simulink model "microgridbelbic"  (R2019a)
settings: Solver=VariableStepAuto  StartTime=0.0  StopTime=6  RelTol=1e-3
undefined symbols (not defined in the file): DiscIntNeverNeededParam, fdesignblkfcn, gcbh, Hydride, Metal, Nickel
libraries: powerlib x242, powerlib_extras x28, BELBICtoolbox x4, dsparch4 x1, electricdrivelib x1, simulink x1, sps_avr x1, powerlib_meascontrol x1, re_lib x1
(part 2 of 4)

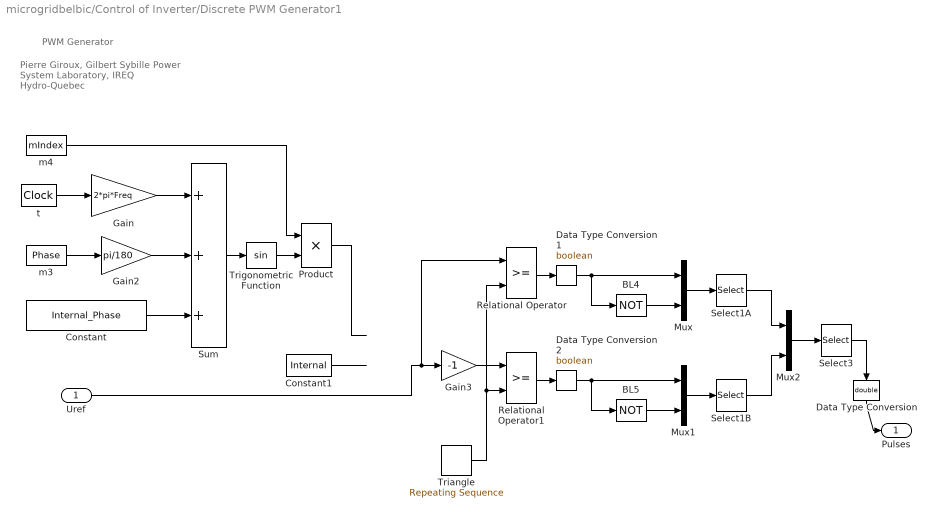
== system microgridbelbic/Control of Inverter/Discrete PWM Generator1 ==
  note: Pierre Giroux, Gilbert Sybille
      | Power System Laboratory, IREQ
      | Hydro-Quebec
  note: PWM Generator
  Uref : Inport
  BL4 : Logic  Operator=NOT  Inputs=1
  BL5 : Logic  Operator=NOT  Inputs=1
  Constant : Constant  Value=Internal_Phase
  Constant1 : Constant  Value=Internal
  Data Type Conversion : DataTypeConversion  OutDataTypeStr=double  SaturateOnIntegerOverflow=on  RndMeth=Zero
  Data Type Conversion1 : DataTypeConversion  OutDataTypeStr=boolean  SaturateOnIntegerOverflow=on  RndMeth=Zero
  Data Type Conversion2 : DataTypeConversion  OutDataTypeStr=boolean  SaturateOnIntegerOverflow=on  RndMeth=Zero
  Gain : Gain  Gain=2*pi*Freq  SaturateOnIntegerOverflow=on  OutDataTypeStr=Inherit: Same as input  ParamDataTypeStr=Inherit: Same as input
  Gain2 : Gain  Gain=pi/180  SaturateOnIntegerOverflow=on  OutDataTypeStr=Inherit: Same as input  ParamDataTypeStr=Inherit: Same as input
  Gain3 : Gain  Gain=-1  SaturateOnIntegerOverflow=on  OutDataTypeStr=Inherit: Same as input  ParamDataTypeStr=Inherit: Same as input
  Mux : Mux  Inputs=2
  Mux1 : Mux  Inputs=2
  Mux2 : Mux  Inputs=2
  Product : Product  SaturateOnIntegerOverflow=on  InputSameDT=on  OutDataTypeStr=Inherit: Same as first input
  Relational Operator : RelationalOperator  RndMeth=Nearest  InputSameDT=on
  Relational Operator1 : RelationalOperator  RndMeth=Nearest  InputSameDT=on
  Select1A : Selector  InputPortWidth=Select1_PortWidth  IndexOptions=Index vector (dialog)  Indices=Select1_Elements  OutputSizes=1
  Select1B : Selector  InputPortWidth=Select1_PortWidth  IndexOptions=Index vector (dialog)  Indices=Select1_Elements  OutputSizes=1
  Select3 : Selector  InputPortWidth=Select3_PortWidth  IndexOptions=Index vector (dialog)  Indices=Select3_Elements  OutputSizes=1
  Sum : Sum  Inputs=+++  SaturateOnIntegerOverflow=on  InputSameDT=on  OutDataTypeStr=Inherit: Same as first input
  Triangle : simulink/Sources/Repeating Sequence  rep_seq_t=[0 1/Fc/4 3/Fc/4 1/Fc]  rep_seq_y=[0 -1 1 0]
  Trigonometric Function : Trigonometry
  m3 : Constant  Value=Phase
  m4 : Constant  Value=mIndex
  t : DigitalClock  SampleTime=Ts
  Pulses : Outport
  wires:
  Mux2/1 -> Select3/1
  Select1B/1 -> Mux2/2
  Select1A/1 -> Mux2/1
  Mux1/1 -> Select1B/1
  Mux/1 -> Select1A/1
  BL5/1 -> Mux1/2
  BL4/1 -> Mux/2
  Gain3/1 -> Relational Operator1/1
  Triangle/1 -> Relational Operator1/2, Relational Operator/2
  Product/1 -> ?
  Constant1/1 -> ?
  Uref/1 -> Relational Operator/1, Gain3/1
  Trigonometric Function/1 -> Product/2
  Sum/1 -> Trigonometric Function/1
  m4/1 -> Product/1
  Constant/1 -> Sum/3
  m3/1 -> Gain2/1
  Gain2/1 -> Sum/2
  Gain/1 -> Sum/1
  t/1 -> Gain/1
  Select3/1 -> Data Type Conversion/1
  Data Type Conversion/1 -> Pulses/1
  Relational Operator/1 -> Data Type Conversion1/1
  Data Type Conversion1/1 -> BL4/1, Mux/1
  Relational Operator1/1 -> Data Type Conversion2/1
  Data Type Conversion2/1 -> BL5/1, Mux1/1

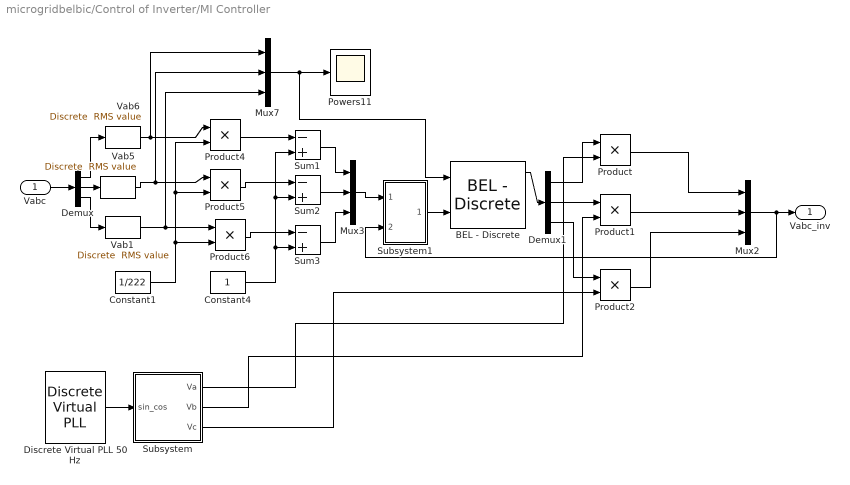
== system microgridbelbic/Control of Inverter/MI Controller ==
  Vabc : Inport
  BEL - Discrete : BELBICtoolbox/Discrete-time/BEL - Discrete  alfa=0.001  beta=0.008  V=0.99  Vth=0.099  W=0.1  T=1
      settings: SourceProductName=BELBIC Toolbox
  Constant1 : Constant  Value=1/222
  Constant4 : Constant
  Demux : Demux  Outputs=3
  Demux1 : Demux  Outputs=3
  Discrete Virtual PLL 50 Hz : powerlib_extras/Discrete  Control Blocks/Discrete Virtual PLL  Freq=50  Phase=0  Ts=20e-6
      settings: SourceProductName=Simscape Electrical  SourceProductBaseCode=PS
  Mux2 : Mux  Inputs=3
  Mux3 : Mux  Inputs=3
  Mux7 : Mux  Inputs=3
  Powers11 : Scope
  Product{,1..2,4..6} (6 alike) : Product  RndMeth=Zero
  Subsystem : Subsystem
  Subsystem1 : Subsystem
  Sum1 : Sum  Inputs=-+  SaturateOnIntegerOverflow=on  InputSameDT=on  OutDataTypeStr=Inherit: Same as first input
  Sum2 : Sum  Inputs=-+  SaturateOnIntegerOverflow=on  InputSameDT=on  OutDataTypeStr=Inherit: Same as first input
  Sum3 : Sum  Inputs=-+  SaturateOnIntegerOverflow=on  InputSameDT=on  OutDataTypeStr=Inherit: Same as first input
  Vab1 : powerlib_extras/Discrete Measurements/Discrete  RMS value  Freq=50  Mag_Init=0  Ts=20e-6
      settings: SourceProductName=Simscape Electrical  SourceProductBaseCode=PS
  Vab5 : powerlib_extras/Discrete Measurements/Discrete  RMS value  Freq=50  Mag_Init=0  Ts=20e-6
      settings: SourceProductName=Simscape Electrical  SourceProductBaseCode=PS
  Vab6 : powerlib_extras/Discrete Measurements/Discrete  RMS value  Freq=50  Mag_Init=0  Ts=20e-6
      settings: SourceProductName=Simscape Electrical  SourceProductBaseCode=PS
  Vabc_inv : Outport
  wires:
  Mux2/1 -> Subsystem1/2(In2), Vabc_inv/1
  Product/1 -> Mux2/1
  Product1/1 -> Mux2/2
  Product2/1 -> Mux2/3
  Vab5/1 -> Mux7/2, Product5/1
  Vab1/1 -> Mux7/3, Product6/1
  Constant4/1 -> Sum3/2, Sum2/2, Sum1/2
  Sum1/1 -> Mux3/1
  Vabc/1 -> Demux/1
  Demux/1 -> Vab6/1
  Demux/2 -> Vab5/1
  Demux/3 -> Vab1/1
  Sum2/1 -> Mux3/2
  Sum3/1 -> Mux3/3
  Demux1/1 -> Product/1
  Demux1/2 -> Product1/1
  Demux1/3 -> Product2/1
  Product4/1 -> Sum1/1
  Product5/1 -> Sum2/1
  Product6/1 -> Sum3/1
  Vab6/1 -> Mux7/1, Product4/1
  Mux7/1 -> BEL - Discrete/1, Powers11/1
  Discrete Virtual PLL 50 Hz/2 -> Subsystem/1(sin_cos)
  Subsystem/1(Va) -> Product/2
  Subsystem/2(Vb) -> Product1/2
  Subsystem/3(Vc) -> Product2/2
  Constant1/1 -> Product6/2, Product5/2, Product4/2
  BEL - Discrete/1 -> Demux1/1
  Mux3/1 -> Subsystem1/1(In1)
  Subsystem1/1(Out1) -> BEL - Discrete/2

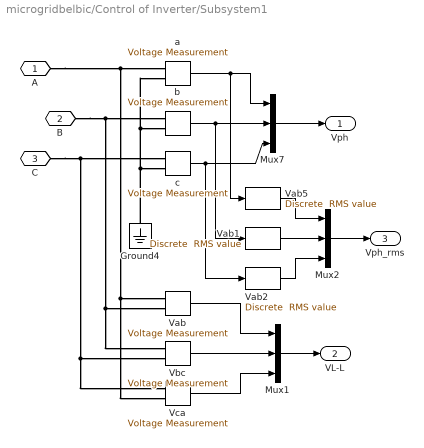
== system microgridbelbic/Control of Inverter/Subsystem1 ==
  Ground4 : powerlib/Elements/Ground  LConnTagsString=a
      settings: SourceProductName=Simscape Electrical
  Mux1 : Mux  Inputs=3
  Mux2 : Mux  Inputs=3
  Mux7 : Mux  Inputs=3
  Vab : powerlib/Measurements/Voltage Measurement  Tag=PoWeRsYsTeMmEaSuReMeNt  PhasorSimulation=off  OutputType=Magnitude  PSBequivalent=0
      settings: SourceProductName=Simscape Electrical
  Vab1 : powerlib_extras/Discrete Measurements/Discrete  RMS value  Freq=50  Mag_Init=0  Ts=20e-6
      settings: SourceProductName=Simscape Electrical  SourceProductBaseCode=PS
  Vab2 : powerlib_extras/Discrete Measurements/Discrete  RMS value  Freq=50  Mag_Init=0  Ts=20e-6
      settings: SourceProductName=Simscape Electrical  SourceProductBaseCode=PS
  Vab5 : powerlib_extras/Discrete Measurements/Discrete  RMS value  Freq=50  Mag_Init=0  Ts=20e-6
      settings: SourceProductName=Simscape Electrical  SourceProductBaseCode=PS
  Vbc : powerlib/Measurements/Voltage Measurement  Tag=PoWeRsYsTeMmEaSuReMeNt  PhasorSimulation=off  OutputType=Magnitude  PSBequivalent=0
      settings: SourceProductName=Simscape Electrical
  Vca : powerlib/Measurements/Voltage Measurement  Tag=PoWeRsYsTeMmEaSuReMeNt  PhasorSimulation=off  OutputType=Magnitude  PSBequivalent=0
      settings: SourceProductName=Simscape Electrical
  a : powerlib/Measurements/Voltage Measurement  Tag=PoWeRsYsTeMmEaSuReMeNt  PhasorSimulation=off  OutputType=Magnitude  PSBequivalent=0
      settings: SourceProductName=Simscape Electrical
  b : powerlib/Measurements/Voltage Measurement  Tag=PoWeRsYsTeMmEaSuReMeNt  PhasorSimulation=off  OutputType=Magnitude  PSBequivalent=0
      settings: SourceProductName=Simscape Electrical
  c : powerlib/Measurements/Voltage Measurement  Tag=PoWeRsYsTeMmEaSuReMeNt  PhasorSimulation=off  OutputType=Magnitude  PSBequivalent=0
      settings: SourceProductName=Simscape Electrical
  A : PMIOPort  Side=Left
  B : PMIOPort  Port=2  Side=Left
  C : PMIOPort  Port=3  Side=Left
  Vph : Outport
  VL-L : Outport  Port=2
  Vph_rms : Outport  Port=3
  wires:
  a/1 -> Mux7/1, Vab5/1
  b/1 -> Mux7/2, Vab1/1
  c/1 -> Mux7/3, Vab2/1
  Mux7/1 -> Vph/1
  Vab/1 -> Mux1/1
  Vbc/1 -> Mux1/2
  Vca/1 -> Mux1/3
  Mux1/1 -> VL-L/1
  Vab5/1 -> Mux2/1
  Vab1/1 -> Mux2/2
  Vab2/1 -> Mux2/3
  Mux2/1 -> Vph_rms/1
  connections:
  Ground4/LConn1 -- c/LConn2 -- b/LConn2 -- a/LConn2
  A/RConn1 -- a/LConn1 -- Vab/LConn1 -- Vca/LConn2
  B/RConn1 -- b/LConn1 -- Vab/LConn2 -- Vbc/LConn1
  C/RConn1 -- c/LConn1 -- Vbc/LConn2 -- Vca/LConn1

== system microgridbelbic/Diesel/Diesel Engine Speed & Voltage Control ==
  wref : Inport
  Vtref : Inport  Port=2
  m : Inport  Port=3
  Bus Selector : BusSelector  OutputSignals="Mechanical.Rotor speed  wm  (pu)"
  Bus Selector1 : BusSelector  OutputSignals="dq0 components.Stator voltage  vd (pu),dq0 components.Stator voltage  vq (pu)"  OutputAsBus=on
  Demux2 : Demux  Outputs=2
  EXCITATION : sps_avr/Excitation System  tr=20e-3  reg=[ 200, 0.02 ]  exc=[ 1, 0 ]  tgr=[ 0, 0 ]  damp=[ 0.001, 0.1 ]  sat=[ 0, 0 ]  lim=[ 0, 6, 0 ]  v0=[1,1.42734]
      settings: SourceProductName=Simscape Electrical  SourceProductBaseCode=PS
  Fcn : Fcn  Expr=sqrt(u(1)^2 + u(2)^2)
  GOVERNOR & DIESEL ENGINE : Subsystem  mask(Diesel Engine & Governor){K=40, Tr=[0.01 0.02 0.2], Ta=[0.25 0.009 0.0384], Tlim=[0 1.1], Td=0.024, Pm0=0.000270147}
      mask prompts: K "Regulator gain K:"; Tr "Regulator time constants [T1 T2 T3 ] (s) :"; Ta "Actuator time constants [T4 T5 T6] (s) :"; Tlim "Torque limits [Tmin Tmax] (pu) :"; Td "Engine time delay Td (s) :"; Pm0 "Initial value of mechanical power  Pm0 (pu) :"
      mask help:
      | This block implements a diesel engine and governor system:
      | 1st and 2nd inputs: Desired and actual speed (pu)
      | Output: Diesel engine mechanical power.Motor inertia should be combined with generator.
      | Controller transfer function:
      |      Hc=K.(1+T3.s)/(1+T1.s+T1.T2.s^2)
      | Actuator transfer function :
      |      Ha= (1+T4.s) / [ (s (1+T5.s)(1+T6.s) ]
      | Motor :
      |      Time delay Td
      |
      | (See reference in Tutorial Session 5)
  Ground : Ground
  Pm : Outport  InitialOutput=0
  Vf : Outport  Port=2  InitialOutput=0
  Vt : Outport  Port=3  InitialOutput=0
  w : Outport  Port=4  InitialOutput=0
  wires:
  Ground/1 -> EXCITATION/4
  m/1 -> Bus Selector/1, Bus Selector1/1
  wref/1 -> GOVERNOR & DIESEL ENGINE/1(wref (pu))
  Demux2/2 -> EXCITATION/3
  EXCITATION/1 -> Vf/1
  GOVERNOR & DIESEL ENGINE/1(Pmec (pu)) -> Pm/1
  Vtref/1 -> EXCITATION/1
  Demux2/1 -> EXCITATION/2
  Bus Selector1/1 -> Demux2/1, Fcn/1
  Fcn/1 -> Vt/1
  Bus Selector/1 -> GOVERNOR & DIESEL ENGINE/2(w (pu)), w/1  "<Rotor speed  wm  (pu)>"

== system microgridbelbic/Subsystem/Subsystem ==
  In1 : Inport
  In2 : Inport  Port=2
  Add : Sum
  Gain1 : Gain  Gain=0.02
  Gain2 : Gain  Gain=0.001
  Out1 : Outport
  wires:
  In1/1 -> Gain1/1
  Gain2/1 -> Add/2
  In2/1 -> Gain2/1
  Add/1 -> Out1/1
  Gain1/1 -> Add/1

== system microgridbelbic/Subsystem1/Subsystem ==
  In1 : Inport
  array1 : Subsystem
  array6 : Subsystem
  array7 : Subsystem
  Conn3 : PMIOPort  Side=Right
  Conn4 : PMIOPort  Port=2  Side=Right
  wires:
  In1/1 -> array1/1(In1), array7/1(In1), array6/1(In1)
  connections:
  array1/RConn2 -- array6/RConn2 -- array7/RConn2 -- Conn4/RConn1
  array1/RConn1 -- array6/RConn1 -- array7/RConn1 -- Conn3/RConn1

== system microgridbelbic/Subsystem1/Subsystem1 ==
  In1 : Inport
  array1 : Subsystem
  array6 : Subsystem
  array7 : Subsystem
  Conn3 : PMIOPort  Side=Right
  Conn4 : PMIOPort  Port=2  Side=Right
  wires:
  In1/1 -> array1/1(In1), array7/1(In1), array6/1(In1)
  connections:
  array1/RConn1 -- array7/RConn1 -- array6/RConn1 -- Conn3/RConn1
  array1/RConn2 -- array7/RConn2 -- array6/RConn2 -- Conn4/RConn1

== system microgridbelbic/Subsystem1/Subsystem2 ==
  In1 : Inport
  array1 : Subsystem
  array6 : Subsystem
  array7 : Subsystem
  Conn3 : PMIOPort  Side=Right
  Conn4 : PMIOPort  Port=2  Side=Right
  wires:
  In1/1 -> array1/1(In1), array7/1(In1), array6/1(In1)
  connections:
  array1/RConn2 -- array7/RConn2 -- array6/RConn2 -- Conn4/RConn1
  array1/RConn1 -- array7/RConn1 -- array6/RConn1 -- Conn3/RConn1

== system microgridbelbic/Subsystem1/Subsystem3 ==
  In1 : Inport
  array1 : Subsystem
  array6 : Subsystem
  array7 : Subsystem
  Conn3 : PMIOPort  Side=Right
  Conn4 : PMIOPort  Port=2  Side=Right
  wires:
  In1/1 -> array1/1(In1), array7/1(In1), array6/1(In1)
  connections:
  array1/RConn2 -- array7/RConn2 -- array6/RConn2 -- Conn4/RConn1
  array1/RConn1 -- array7/RConn1 -- array6/RConn1 -- Conn3/RConn1

== system microgridbelbic/Subsystem1/Subsystem4 ==
  In1 : Inport
  array1 : Subsystem
  array6 : Subsystem
  array7 : Subsystem
  Conn3 : PMIOPort  Side=Right
  Conn4 : PMIOPort  Port=2  Side=Right
  wires:
  In1/1 -> array1/1(In1), array7/1(In1), array6/1(In1)
  connections:
  array1/RConn1 -- array7/RConn1 -- Conn3/RConn1 -- array6/RConn1
  array1/RConn2 -- array7/RConn2 -- Conn4/RConn1 -- array6/RConn2

== system microgridbelbic/Wind pulses/Current Controller1 ==
  Iref : Inport
  Ia : Inport  Port=2
  Relay : Relay  OnSwitchValue=h/2  OffSwitchValue=-h/2
  Sum1 : Sum  Inputs=-+  SaturateOnIntegerOverflow=on  InputSameDT=on  OutDataTypeStr=Inherit: Same as first input
  g : Outport  InitialOutput=0
  error1 : Outport  Port=2  InitialOutput=0
  wires:
  Sum1/1 -> error1/1, Relay/1
  Iref/1 -> Sum1/2
  Ia/1 -> Sum1/1
  Relay/1 -> g/1

== system microgridbelbic/Wind pulses/Subsystem ==
  Tref : Inport
  wm : Inport  Port=2
  Vd : Inport  Port=3
  Avoid division by zero : Saturate  UpperLimit=1e6  LowerLimit=1e-6
  Base Torque1 : Product  Inputs=*/  RndMeth=Zero
  Product1 : Product  RndMeth=Zero
  Id_ref : Outport
  wires:
  Vd/1 -> Avoid division by zero/1
  Base Torque1/1 -> Id_ref/1
  wm/1 -> Product1/2
  Tref/1 -> Product1/1
  Avoid division by zero/1 -> Base Torque1/2
  Product1/1 -> Base Torque1/1

== system microgridbelbic/Wind pulses/Torque reference 1 ==
  wm : Inport
  1\ib1 : Gain  Gain=0.001189  SaturateOnIntegerOverflow=on  OutDataTypeStr=Inherit: Same as input  ParamDataTypeStr=Inherit: Same as input
  1\ib2 : Gain  Gain=0.0197  SaturateOnIntegerOverflow=on  OutDataTypeStr=Inherit: Same as input  ParamDataTypeStr=Inherit: Same as input
  Add : Sum
  Constant2 : Constant  Value=1.791e-3
  Differentiator Filter : Subsystem  DialogController=fdesignblkfcn  InitFcn=fdesignblkfcn(gcbh, {'InitFcn'});  mask(Differentiator Filter){}
      mask help: Design a differentiator filter
      settings: CopyFcn=fdesignblkfcn(gcbh, {'CopyFcn'});
      mask Help: helpview(mapfilelocation('dspblks'), 'dspdifferentiatorfilter')
      mask Display: disp('Differentiator');
  Math Function : Math  Operator=square  SaturateOnIntegerOverflow=on
  Product1 : Product  RndMeth=Zero
  Ref. sat.1 : Saturate  UpperLimit=inf  LowerLimit=0
  Subtract : Sum  Inputs=+-
  Tref : Outport
  wires:
  Subtract/1 -> Ref. sat.1/1
  1\ib2/1 -> Add/1
  Product1/1 -> Subtract/1
  1\ib1/1 -> Add/2
  Differentiator Filter/1(Out) -> 1\ib2/1
  Ref. sat.1/1 -> Tref/1
  wm/1 -> 1\ib1/1, Differentiator Filter/1(In), Math Function/1
  Constant2/1 -> Product1/2
  Math Function/1 -> Product1/1

== system microgridbelbic/wind1 20.1KW/Pitch_angle-controller ==
  wr : Inport
  0-pitch_max : Saturate  UpperLimit=45  LowerLimit=0
  Constant2 : Constant
  "Rate Limiter   " : RateLimiter  RisingSlewLimit=2  FallingSlewLimit=-2
  Sum : Sum  Inputs=|+-  SaturateOnIntegerOverflow=on
  genertaor terminal6 : Scope  NumInputPorts=2
  pitch_gain : Gain  Gain=500  SaturateOnIntegerOverflow=on  OutDataTypeStr=Inherit: Same as input  ParamDataTypeStr=Inherit: Same as input
  Pitch_angle : Outport
  wires:
  wr/1 -> Sum/1
  0-pitch_max/1 -> genertaor terminal6/2, "Rate Limiter   "/1
  Constant2/1 -> Sum/2
  Sum/1 -> pitch_gain/1
  pitch_gain/1 -> 0-pitch_max/1
  "Rate Limiter   "/1 -> genertaor terminal6/1, Pitch_angle/1

== system microgridbelbic/Control of Inverter/MI Controller/Subsystem ==
  sin_cos : Inport  PortDimensions=2
  Demux : Demux  Outputs=2
  Fcn2 : Fcn  Expr=1*u[1]
  Fcn4 : Fcn  Expr=1*u[3]
  Fcn5 : Fcn  Expr=1*u[5]
  K1 : Constant  Value=0.5
  K2 : Constant  Value=sqrt(3)/2
  Mux2 : Mux  Inputs=6
  Product{,1..3} (4 alike) : Product  SaturateOnIntegerOverflow=on  InputSameDT=on  OutDataTypeStr=Inherit: Same as first input
  Sum : Sum  Inputs=--  SaturateOnIntegerOverflow=on  InputSameDT=on  OutDataTypeStr=Inherit: Same as first input
  Sum1 : Sum  Inputs=-+  SaturateOnIntegerOverflow=on  InputSameDT=on  OutDataTypeStr=Inherit: Same as first input
  Sum2 : Sum  Inputs=--  SaturateOnIntegerOverflow=on  InputSameDT=on  OutDataTypeStr=Inherit: Same as first input
  Sum3 : Sum  Inputs=--  SaturateOnIntegerOverflow=on  InputSameDT=on  OutDataTypeStr=Inherit: Same as first input
  Va : Outport
  Vb : Outport  Port=2
  Vc : Outport  Port=3
  wires:
  sin_cos/1 -> Demux/1
  Demux/1 -> Product/1, Product2/1, Sum2/2, Mux2/1  "sin(wt)"
  Product/1 -> Sum/1
  Product1/1 -> Sum/2
  Product3/1 -> Sum1/1
  Product2/1 -> Sum1/2
  Sum3/1 -> Mux2/6  "cos(wt+2pi/3)"
  Sum2/1 -> Mux2/5  "sin(wt+2pi/3)"
  K1/1 -> Product/2, Product3/2
  K2/1 -> Product1/2, Product2/2
  Sum/1 -> Mux2/3, Sum2/1  "sin(wt-2pi/3)"
  Sum1/1 -> Mux2/4, Sum3/1  "cos(wt-2pi/3)"
  Demux/2 -> Sum3/2, Product3/1, Product1/1, Mux2/2  "cos(wt)"
  Mux2/1 -> Fcn2/1, Fcn4/1, Fcn5/1
  Fcn2/1 -> Va/1
  Fcn4/1 -> Vb/1
  Fcn5/1 -> Vc/1

== system microgridbelbic/Control of Inverter/MI Controller/Subsystem1 ==
  In1 : Inport
  In2 : Inport  Port=2
  Add : Sum
  Gain1 : Gain  Gain=0.9
  Gain2 : Gain  Gain=0.01
  Out1 : Outport
  wires:
  In1/1 -> Gain1/1
  Gain2/1 -> Add/2
  In2/1 -> Gain2/1
  Add/1 -> Out1/1
  Gain1/1 -> Add/1

== system microgridbelbic/Diesel/Diesel Engine Speed & Voltage Control/GOVERNOR & DIESEL ENGINE ==
  note: ACTUATOR
  wref (pu) : Inport
  w (pu) : Inport  Port=2
  CONTROL SYSTEM : TransferFcn  Numerator=([Tr(3) 1])  Denominator="([Tr(1)*Tr(2)  Tr(1) 1])"
  ENGINE Td : TransportDelay  DelayTime=Td  InitialOutput=Pm0
  Gain K : Gain  Gain=K  SaturateOnIntegerOverflow=on  OutDataTypeStr=Inherit: Same as input  ParamDataTypeStr=Inherit: Same as input
  Integrator : Integrator  InitialCondition=Pm0  LimitOutput=on  UpperSaturationLimit=Tlim(2)  LowerSaturationLimit=Tlim(1)
  Product : Product  SaturateOnIntegerOverflow=on  InputSameDT=on  OutDataTypeStr=Inherit: Same as first input
  Sum : Sum  Inputs=+-  SaturateOnIntegerOverflow=on  InputSameDT=on  OutDataTypeStr=Inherit: Same as first input
  TF1 : TransferFcn  Numerator=([Ta(1) 1])  Denominator=([Ta(2) 1])
  TF2 : TransferFcn  Numerator=1  Denominator=([Ta(3) 1])
  Pmec (pu) : Outport  InitialOutput=0
  wires:
  Gain K/1 -> TF1/1
  Sum/1 -> CONTROL SYSTEM/1
  CONTROL SYSTEM/1 -> Gain K/1
  TF1/1 -> TF2/1
  w (pu)/1 -> Product/2, Sum/2
  ENGINE Td/1 -> Product/1
  wref (pu)/1 -> Sum/1
  Product/1 -> Pmec (pu)/1
  TF2/1 -> Integrator/1
  Integrator/1 -> ENGINE Td/1  "Torque"

== system microgridbelbic/Subsystem1/Subsystem/array1 ==
  In1 : Inport
  Solar : Subsystem
  Conn1 : PMIOPort  Side=Right
  Conn2 : PMIOPort  Port=2  Side=Right
  wires:
  In1/1 -> Solar/1(In1)
  connections:
  Solar/RConn1 -- Conn1/RConn1
  Solar/RConn3 -- Solar/RConn2
  Conn2/RConn1 -- Solar/RConn4

== system microgridbelbic/Subsystem1/Subsystem/array6 ==
  In1 : Inport
  Solar : Subsystem
  Conn1 : PMIOPort  Side=Right
  Conn2 : PMIOPort  Port=2  Side=Right
  wires:
  In1/1 -> Solar/1(In1)
  connections:
  Conn2/RConn1 -- Solar/RConn4
  Solar/RConn3 -- Solar/RConn2
  Solar/RConn1 -- Conn1/RConn1

== system microgridbelbic/Subsystem1/Subsystem/array7 ==
  In1 : Inport
  Solar : Subsystem
  Conn1 : PMIOPort  Side=Right
  Conn2 : PMIOPort  Port=2  Side=Right
  wires:
  In1/1 -> Solar/1(In1)
  connections:
  Conn2/RConn1 -- Solar/RConn4
  Solar/RConn3 -- Solar/RConn2
  Solar/RConn1 -- Conn1/RConn1

== system microgridbelbic/Subsystem1/Subsystem1/array1 ==
  In1 : Inport
  Solar : Subsystem
  Conn1 : PMIOPort  Side=Right
  Conn2 : PMIOPort  Port=2  Side=Right
  wires:
  In1/1 -> Solar/1(In1)
  connections:
  Conn2/RConn1 -- Solar/RConn4
  Solar/RConn3 -- Solar/RConn2
  Solar/RConn1 -- Conn1/RConn1

== system microgridbelbic/Subsystem1/Subsystem1/array6 ==
  In1 : Inport
  Solar : Subsystem
  Conn1 : PMIOPort  Side=Right
  Conn2 : PMIOPort  Port=2  Side=Right
  wires:
  In1/1 -> Solar/1(In1)
  connections:
  Solar/RConn1 -- Conn1/RConn1
  Solar/RConn3 -- Solar/RConn2
  Conn2/RConn1 -- Solar/RConn4

== system microgridbelbic/Subsystem1/Subsystem1/array7 ==
  In1 : Inport
  Solar : Subsystem
  Conn1 : PMIOPort  Side=Right
  Conn2 : PMIOPort  Port=2  Side=Right
  wires:
  In1/1 -> Solar/1(In1)
  connections:
  Solar/RConn1 -- Conn1/RConn1
  Solar/RConn3 -- Solar/RConn2
  Conn2/RConn1 -- Solar/RConn4

== system microgridbelbic/Subsystem1/Subsystem2/array1 ==
  In1 : Inport
  Solar : Subsystem
  Conn1 : PMIOPort  Side=Right
  Conn2 : PMIOPort  Port=2  Side=Right
  wires:
  In1/1 -> Solar/1(In1)
  connections:
  Solar/RConn1 -- Conn1/RConn1
  Solar/RConn3 -- Solar/RConn2
  Conn2/RConn1 -- Solar/RConn4

== system microgridbelbic/Subsystem1/Subsystem2/array6 ==
  In1 : Inport
  Solar : Subsystem
  Conn1 : PMIOPort  Side=Right
  Conn2 : PMIOPort  Port=2  Side=Right
  wires:
  In1/1 -> Solar/1(In1)
  connections:
  Conn2/RConn1 -- Solar/RConn4
  Solar/RConn3 -- Solar/RConn2
  Solar/RConn1 -- Conn1/RConn1

== system microgridbelbic/Subsystem1/Subsystem2/array7 ==
  In1 : Inport
  Solar : Subsystem
  Conn1 : PMIOPort  Side=Right
  Conn2 : PMIOPort  Port=2  Side=Right
  wires:
  In1/1 -> Solar/1(In1)
  connections:
  Conn2/RConn1 -- Solar/RConn4
  Solar/RConn3 -- Solar/RConn2
  Solar/RConn1 -- Conn1/RConn1

== system microgridbelbic/Subsystem1/Subsystem3/array1 ==
  In1 : Inport
  Solar : Subsystem
  Conn1 : PMIOPort  Side=Right
  Conn2 : PMIOPort  Port=2  Side=Right
  wires:
  In1/1 -> Solar/1(In1)
  connections:
  Solar/RConn1 -- Conn1/RConn1
  Solar/RConn3 -- Solar/RConn2
  Conn2/RConn1 -- Solar/RConn4

== system microgridbelbic/Subsystem1/Subsystem3/array6 ==
  In1 : Inport
  Solar : Subsystem
  Conn1 : PMIOPort  Side=Right
  Conn2 : PMIOPort  Port=2  Side=Right
  wires:
  In1/1 -> Solar/1(In1)
  connections:
  Conn2/RConn1 -- Solar/RConn4
  Solar/RConn3 -- Solar/RConn2
  Solar/RConn1 -- Conn1/RConn1

== system microgridbelbic/Subsystem1/Subsystem3/array7 ==
  In1 : Inport
  Solar : Subsystem
  Conn1 : PMIOPort  Side=Right
  Conn2 : PMIOPort  Port=2  Side=Right
  wires:
  In1/1 -> Solar/1(In1)
  connections:
  Conn2/RConn1 -- Solar/RConn4
  Solar/RConn3 -- Solar/RConn2
  Solar/RConn1 -- Conn1/RConn1

== system microgridbelbic/Subsystem1/Subsystem4/array1 ==
  In1 : Inport
  Solar : Subsystem
  Conn1 : PMIOPort  Side=Right
  Conn2 : PMIOPort  Port=2  Side=Right
  wires:
  In1/1 -> Solar/1(In1)
  connections:
  Conn2/RConn1 -- Solar/RConn4
  Solar/RConn3 -- Solar/RConn2
  Solar/RConn1 -- Conn1/RConn1

== system microgridbelbic/Subsystem1/Subsystem4/array6 ==
  In1 : Inport
  Solar : Subsystem
  Conn1 : PMIOPort  Side=Right
  Conn2 : PMIOPort  Port=2  Side=Right
  wires:
  In1/1 -> Solar/1(In1)
  connections:
  Solar/RConn1 -- Conn1/RConn1
  Solar/RConn3 -- Solar/RConn2
  Conn2/RConn1 -- Solar/RConn4

== system microgridbelbic/Subsystem1/Subsystem4/array7 ==
  In1 : Inport
  Solar : Subsystem
  Conn1 : PMIOPort  Side=Right
  Conn2 : PMIOPort  Port=2  Side=Right
  wires:
  In1/1 -> Solar/1(In1)
  connections:
  Solar/RConn1 -- Conn1/RConn1
  Solar/RConn3 -- Solar/RConn2
  Conn2/RConn1 -- Solar/RConn4

== system microgridbelbic/Wind pulses/Torque reference 1/Differentiator Filter ==
  In : Inport
  Generated Filter Block : Subsystem  Tag=FilterWizardSubSystem
      settings: ErrorFcn=dspFilterRealizedInBasicElemsAlgLoopErrFcnCallback
  Out : Outport
  wires:
  In/1 -> Generated Filter Block/1(Input)
  Generated Filter Block/1(Output) -> Out/1

== system microgridbelbic/Subsystem1/Subsystem/array1/Solar ==
  In1 : Inport
  Subsystem1 : Subsystem
  Subsystem5 : Subsystem
  1 : PMIOPort  Tag=PMCPort  Side=Right
  2 : PMIOPort  Tag=PMCPort  Port=2  Side=Right
  3 : PMIOPort  Tag=PMCPort  Port=3  Side=Right
  4 : PMIOPort  Tag=PMCPort  Port=4  Side=Right
  wires:
  In1/1 -> Subsystem1/1(In1), Subsystem5/1(In1)
  connections:
  3/RConn1 -- Subsystem1/RConn1
  4/RConn1 -- Subsystem1/RConn2
  1/RConn1 -- Subsystem5/RConn1
  2/RConn1 -- Subsystem5/RConn2

== system microgridbelbic/Subsystem1/Subsystem/array6/Solar ==
  In1 : Inport
  "11= Vmpp=336V, Voc=406V" : Subsystem
  "11=336V, 406 V" : Subsystem
  1 : PMIOPort  Tag=PMCPort  Side=Right
  2 : PMIOPort  Tag=PMCPort  Port=2  Side=Right
  3 : PMIOPort  Tag=PMCPort  Port=3  Side=Right
  4 : PMIOPort  Tag=PMCPort  Port=4  Side=Right
  wires:
  In1/1 -> "11= Vmpp=336V, Voc=406V"/1(In1), "11=336V, 406 V"/1(In1)
  connections:
  2/RConn1 -- "11= Vmpp=336V, Voc=406V"/RConn2
  1/RConn1 -- "11= Vmpp=336V, Voc=406V"/RConn1
  4/RConn1 -- "11=336V, 406 V"/RConn2
  3/RConn1 -- "11=336V, 406 V"/RConn1

== system microgridbelbic/Subsystem1/Subsystem/array7/Solar ==
  In1 : Inport
  Subsystem1 : Subsystem
  Subsystem5 : Subsystem
  1 : PMIOPort  Tag=PMCPort  Side=Right
  2 : PMIOPort  Tag=PMCPort  Port=2  Side=Right
  3 : PMIOPort  Tag=PMCPort  Port=3  Side=Right
  4 : PMIOPort  Tag=PMCPort  Port=4  Side=Right
  wires:
  In1/1 -> Subsystem5/1(In1), Subsystem1/1(In1)
  connections:
  2/RConn1 -- Subsystem5/RConn2
  1/RConn1 -- Subsystem5/RConn1
  4/RConn1 -- Subsystem1/RConn2
  3/RConn1 -- Subsystem1/RConn1

== system microgridbelbic/Subsystem1/Subsystem1/array1/Solar ==
  In1 : Inport
  Subsystem1 : Subsystem
  Subsystem5 : Subsystem
  1 : PMIOPort  Tag=PMCPort  Side=Right
  2 : PMIOPort  Tag=PMCPort  Port=2  Side=Right
  3 : PMIOPort  Tag=PMCPort  Port=3  Side=Right
  4 : PMIOPort  Tag=PMCPort  Port=4  Side=Right
  wires:
  In1/1 -> Subsystem5/1(In1), Subsystem1/1(In1)
  connections:
  2/RConn1 -- Subsystem5/RConn2
  1/RConn1 -- Subsystem5/RConn1
  4/RConn1 -- Subsystem1/RConn2
  3/RConn1 -- Subsystem1/RConn1

== system microgridbelbic/Subsystem1/Subsystem1/array6/Solar ==
  In1 : Inport
  "11= Vmpp=336V, Voc=406V" : Subsystem
  "11=336V, 406 V" : Subsystem
  1 : PMIOPort  Tag=PMCPort  Side=Right
  2 : PMIOPort  Tag=PMCPort  Port=2  Side=Right
  3 : PMIOPort  Tag=PMCPort  Port=3  Side=Right
  4 : PMIOPort  Tag=PMCPort  Port=4  Side=Right
  wires:
  In1/1 -> "11=336V, 406 V"/1(In1), "11= Vmpp=336V, Voc=406V"/1(In1)
  connections:
  3/RConn1 -- "11=336V, 406 V"/RConn1
  4/RConn1 -- "11=336V, 406 V"/RConn2
  1/RConn1 -- "11= Vmpp=336V, Voc=406V"/RConn1
  2/RConn1 -- "11= Vmpp=336V, Voc=406V"/RConn2

== system microgridbelbic/Subsystem1/Subsystem1/array7/Solar ==
  In1 : Inport
  Subsystem1 : Subsystem
  Subsystem5 : Subsystem
  1 : PMIOPort  Tag=PMCPort  Side=Right
  2 : PMIOPort  Tag=PMCPort  Port=2  Side=Right
  3 : PMIOPort  Tag=PMCPort  Port=3  Side=Right
  4 : PMIOPort  Tag=PMCPort  Port=4  Side=Right
  wires:
  In1/1 -> Subsystem1/1(In1), Subsystem5/1(In1)
  connections:
  3/RConn1 -- Subsystem1/RConn1
  4/RConn1 -- Subsystem1/RConn2
  1/RConn1 -- Subsystem5/RConn1
  2/RConn1 -- Subsystem5/RConn2

== system microgridbelbic/Subsystem1/Subsystem2/array1/Solar ==
  In1 : Inport
  Subsystem1 : Subsystem
  Subsystem5 : Subsystem
  1 : PMIOPort  Tag=PMCPort  Side=Right
  2 : PMIOPort  Tag=PMCPort  Port=2  Side=Right
  3 : PMIOPort  Tag=PMCPort  Port=3  Side=Right
  4 : PMIOPort  Tag=PMCPort  Port=4  Side=Right
  wires:
  In1/1 -> Subsystem1/1(In1), Subsystem5/1(In1)
  connections:
  3/RConn1 -- Subsystem1/RConn1
  4/RConn1 -- Subsystem1/RConn2
  1/RConn1 -- Subsystem5/RConn1
  2/RConn1 -- Subsystem5/RConn2

== system microgridbelbic/Subsystem1/Subsystem2/array6/Solar ==
  In1 : Inport
  "11= Vmpp=336V, Voc=406V" : Subsystem
  "11=336V, 406 V" : Subsystem
  1 : PMIOPort  Tag=PMCPort  Side=Right
  2 : PMIOPort  Tag=PMCPort  Port=2  Side=Right
  3 : PMIOPort  Tag=PMCPort  Port=3  Side=Right
  4 : PMIOPort  Tag=PMCPort  Port=4  Side=Right
  wires:
  In1/1 -> "11= Vmpp=336V, Voc=406V"/1(In1), "11=336V, 406 V"/1(In1)
  connections:
  2/RConn1 -- "11= Vmpp=336V, Voc=406V"/RConn2
  1/RConn1 -- "11= Vmpp=336V, Voc=406V"/RConn1
  4/RConn1 -- "11=336V, 406 V"/RConn2
  3/RConn1 -- "11=336V, 406 V"/RConn1

== system microgridbelbic/Subsystem1/Subsystem2/array7/Solar ==
  In1 : Inport
  Subsystem1 : Subsystem
  Subsystem5 : Subsystem
  1 : PMIOPort  Tag=PMCPort  Side=Right
  2 : PMIOPort  Tag=PMCPort  Port=2  Side=Right
  3 : PMIOPort  Tag=PMCPort  Port=3  Side=Right
  4 : PMIOPort  Tag=PMCPort  Port=4  Side=Right
  wires:
  In1/1 -> Subsystem5/1(In1), Subsystem1/1(In1)
  connections:
  2/RConn1 -- Subsystem5/RConn2
  1/RConn1 -- Subsystem5/RConn1
  4/RConn1 -- Subsystem1/RConn2
  3/RConn1 -- Subsystem1/RConn1

== system microgridbelbic/Subsystem1/Subsystem3/array1/Solar ==
  In1 : Inport
  Subsystem1 : Subsystem
  Subsystem5 : Subsystem
  1 : PMIOPort  Tag=PMCPort  Side=Right
  2 : PMIOPort  Tag=PMCPort  Port=2  Side=Right
  3 : PMIOPort  Tag=PMCPort  Port=3  Side=Right
  4 : PMIOPort  Tag=PMCPort  Port=4  Side=Right
  wires:
  In1/1 -> Subsystem1/1(In1), Subsystem5/1(In1)
  connections:
  3/RConn1 -- Subsystem1/RConn1
  4/RConn1 -- Subsystem1/RConn2
  1/RConn1 -- Subsystem5/RConn1
  2/RConn1 -- Subsystem5/RConn2

== system microgridbelbic/Subsystem1/Subsystem3/array6/Solar ==
  In1 : Inport
  "11= Vmpp=336V, Voc=406V" : Subsystem
  "11=336V, 406 V" : Subsystem
  1 : PMIOPort  Tag=PMCPort  Side=Right
  2 : PMIOPort  Tag=PMCPort  Port=2  Side=Right
  3 : PMIOPort  Tag=PMCPort  Port=3  Side=Right
  4 : PMIOPort  Tag=PMCPort  Port=4  Side=Right
  wires:
  In1/1 -> "11= Vmpp=336V, Voc=406V"/1(In1), "11=336V, 406 V"/1(In1)
  connections:
  2/RConn1 -- "11= Vmpp=336V, Voc=406V"/RConn2
  1/RConn1 -- "11= Vmpp=336V, Voc=406V"/RConn1
  4/RConn1 -- "11=336V, 406 V"/RConn2
  3/RConn1 -- "11=336V, 406 V"/RConn1

== system microgridbelbic/Subsystem1/Subsystem3/array7/Solar ==
  In1 : Inport
  Subsystem1 : Subsystem
  Subsystem5 : Subsystem
  1 : PMIOPort  Tag=PMCPort  Side=Right
  2 : PMIOPort  Tag=PMCPort  Port=2  Side=Right
  3 : PMIOPort  Tag=PMCPort  Port=3  Side=Right
  4 : PMIOPort  Tag=PMCPort  Port=4  Side=Right
  wires:
  In1/1 -> Subsystem5/1(In1), Subsystem1/1(In1)
  connections:
  2/RConn1 -- Subsystem5/RConn2
  1/RConn1 -- Subsystem5/RConn1
  4/RConn1 -- Subsystem1/RConn2
  3/RConn1 -- Subsystem1/RConn1

== system microgridbelbic/Subsystem1/Subsystem4/array1/Solar ==
  In1 : Inport
  Subsystem1 : Subsystem
  Subsystem5 : Subsystem
  1 : PMIOPort  Tag=PMCPort  Side=Right
  2 : PMIOPort  Tag=PMCPort  Port=2  Side=Right
  3 : PMIOPort  Tag=PMCPort  Port=3  Side=Right
  4 : PMIOPort  Tag=PMCPort  Port=4  Side=Right
  wires:
  In1/1 -> Subsystem5/1(In1), Subsystem1/1(In1)
  connections:
  2/RConn1 -- Subsystem5/RConn2
  1/RConn1 -- Subsystem5/RConn1
  4/RConn1 -- Subsystem1/RConn2
  3/RConn1 -- Subsystem1/RConn1

== system microgridbelbic/Subsystem1/Subsystem4/array6/Solar ==
  In1 : Inport
  "11= Vmpp=336V, Voc=406V" : Subsystem
  "11=336V, 406 V" : Subsystem
  1 : PMIOPort  Tag=PMCPort  Side=Right
  2 : PMIOPort  Tag=PMCPort  Port=2  Side=Right
  3 : PMIOPort  Tag=PMCPort  Port=3  Side=Right
  4 : PMIOPort  Tag=PMCPort  Port=4  Side=Right
  wires:
  In1/1 -> "11=336V, 406 V"/1(In1), "11= Vmpp=336V, Voc=406V"/1(In1)
  connections:
  3/RConn1 -- "11=336V, 406 V"/RConn1
  4/RConn1 -- "11=336V, 406 V"/RConn2
  1/RConn1 -- "11= Vmpp=336V, Voc=406V"/RConn1
  2/RConn1 -- "11= Vmpp=336V, Voc=406V"/RConn2

== system microgridbelbic/Subsystem1/Subsystem4/array7/Solar ==
  In1 : Inport
  Subsystem1 : Subsystem
  Subsystem5 : Subsystem
  1 : PMIOPort  Tag=PMCPort  Side=Right
  2 : PMIOPort  Tag=PMCPort  Port=2  Side=Right
  3 : PMIOPort  Tag=PMCPort  Port=3  Side=Right
  4 : PMIOPort  Tag=PMCPort  Port=4  Side=Right
  wires:
  In1/1 -> Subsystem1/1(In1), Subsystem5/1(In1)
  connections:
  3/RConn1 -- Subsystem1/RConn1
  4/RConn1 -- Subsystem1/RConn2
  1/RConn1 -- Subsystem5/RConn1
  2/RConn1 -- Subsystem5/RConn2

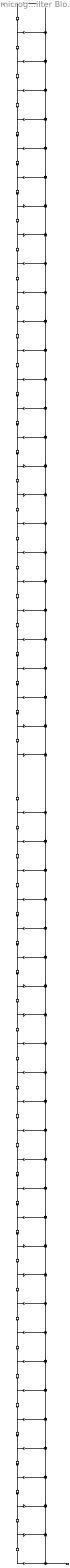
== system microgridbelbic/Wind pulses/Torque reference 1/Differentiator Filter/Generated Filter Block ==
  Input : Inport
  BodyDelay{2..27,30..55} (52 alike) : Delay  DelayLength=1  InitialCondition=0
  BodyDelay29 : Delay  InitialCondition=0
  BodyLSum{2..27,29..55} (53 alike) : Sum  Inputs=++|  SaturateOnIntegerOverflow=on  InputSameDT=on  OutDataTypeStr=Inherit: Same as first input
  b(1) : Gain  Gain=0.0016485839041717864  SaturateOnIntegerOverflow=on  OutDataTypeStr=Inherit: Same as input  ParamDataTypeStr=Inherit: Same as input
  b(10) : Gain  Gain=0.011014879869749052  SaturateOnIntegerOverflow=on  OutDataTypeStr=Inherit: Same as input  ParamDataTypeStr=Inherit: Same as input
  b(11) : Gain  Gain=-0.005763535930488302  SaturateOnIntegerOverflow=on  OutDataTypeStr=Inherit: Same as input  ParamDataTypeStr=Inherit: Same as input
  b(12) : Gain  Gain=-0.0151981830555213  SaturateOnIntegerOverflow=on  OutDataTypeStr=Inherit: Same as input  ParamDataTypeStr=Inherit: Same as input
  b(13) : Gain  Gain=0.0065686388642668125  SaturateOnIntegerOverflow=on  OutDataTypeStr=Inherit: Same as input  ParamDataTypeStr=Inherit: Same as input
  b(14) : Gain  Gain=0.020867949959447688  SaturateOnIntegerOverflow=on  OutDataTypeStr=Inherit: Same as input  ParamDataTypeStr=Inherit: Same as input
  b(15) : Gain  Gain=-0.0070602627960907726  SaturateOnIntegerOverflow=on  OutDataTypeStr=Inherit: Same as input  ParamDataTypeStr=Inherit: Same as input
  b(16) : Gain  Gain=-0.028242635943863115  SaturateOnIntegerOverflow=on  OutDataTypeStr=Inherit: Same as input  ParamDataTypeStr=Inherit: Same as input
  b(17) : Gain  Gain=0.0072704924773104732  SaturateOnIntegerOverflow=on  OutDataTypeStr=Inherit: Same as input  ParamDataTypeStr=Inherit: Same as input
  b(18) : Gain  Gain=0.038329320446368831  SaturateOnIntegerOverflow=on  OutDataTypeStr=Inherit: Same as input  ParamDataTypeStr=Inherit: Same as input
  b(19) : Gain  Gain=-0.0068002265270407491  SaturateOnIntegerOverflow=on  OutDataTypeStr=Inherit: Same as input  ParamDataTypeStr=Inherit: Same as input
  b(2) : Gain  Gain=0.00017042943589110223  SaturateOnIntegerOverflow=on  OutDataTypeStr=Inherit: Same as input  ParamDataTypeStr=Inherit: Same as input
  b(20) : Gain  Gain=-0.052819993002155965  SaturateOnIntegerOverflow=on  OutDataTypeStr=Inherit: Same as input  ParamDataTypeStr=Inherit: Same as input
  b(21) : Gain  Gain=0.0049482783503700268  SaturateOnIntegerOverflow=on  OutDataTypeStr=Inherit: Same as input  ParamDataTypeStr=Inherit: Same as input
  b(22) : Gain  Gain=0.075871674298216826  SaturateOnIntegerOverflow=on  OutDataTypeStr=Inherit: Same as input  ParamDataTypeStr=Inherit: Same as input
  b(23) : Gain  Gain=0.00073312852370662537  SaturateOnIntegerOverflow=on  OutDataTypeStr=Inherit: Same as input  ParamDataTypeStr=Inherit: Same as input
  b(24) : Gain  Gain=-0.11992357305817197  SaturateOnIntegerOverflow=on  OutDataTypeStr=Inherit: Same as input  ParamDataTypeStr=Inherit: Same as input
  b(25) : Gain  Gain=-0.022982436984387535  SaturateOnIntegerOverflow=on  OutDataTypeStr=Inherit: Same as input  ParamDataTypeStr=Inherit: Same as input
  b(26) : Gain  Gain=0.24743192698089667  SaturateOnIntegerOverflow=on  OutDataTypeStr=Inherit: Same as input  ParamDataTypeStr=Inherit: Same as input
  b(27) : Gain  Gain=0.30572927022108953  SaturateOnIntegerOverflow=on  OutDataTypeStr=Inherit: Same as input  ParamDataTypeStr=Inherit: Same as input
  b(29) : Gain  Gain=-0.30572927022108953  SaturateOnIntegerOverflow=on  OutDataTypeStr=Inherit: Same as input  ParamDataTypeStr=Inherit: Same as input
  b(3) : Gain  Gain=-0.0038948238157296179  SaturateOnIntegerOverflow=on  OutDataTypeStr=Inherit: Same as input  ParamDataTypeStr=Inherit: Same as input
  b(30) : Gain  Gain=-0.24743192698089667  SaturateOnIntegerOverflow=on  OutDataTypeStr=Inherit: Same as input  ParamDataTypeStr=Inherit: Same as input
  b(31) : Gain  Gain=0.022982436984387535  SaturateOnIntegerOverflow=on  OutDataTypeStr=Inherit: Same as input  ParamDataTypeStr=Inherit: Same as input
  b(32) : Gain  Gain=0.11992357305817197  SaturateOnIntegerOverflow=on  OutDataTypeStr=Inherit: Same as input  ParamDataTypeStr=Inherit: Same as input
  b(33) : Gain  Gain=-0.00073312852370662537  SaturateOnIntegerOverflow=on  OutDataTypeStr=Inherit: Same as input  ParamDataTypeStr=Inherit: Same as input
  b(34) : Gain  Gain=-0.075871674298216826  SaturateOnIntegerOverflow=on  OutDataTypeStr=Inherit: Same as input  ParamDataTypeStr=Inherit: Same as input
  b(35) : Gain  Gain=-0.0049482783503700268  SaturateOnIntegerOverflow=on  OutDataTypeStr=Inherit: Same as input  ParamDataTypeStr=Inherit: Same as input
  b(36) : Gain  Gain=0.052819993002155965  SaturateOnIntegerOverflow=on  OutDataTypeStr=Inherit: Same as input  ParamDataTypeStr=Inherit: Same as input
  b(37) : Gain  Gain=0.0068002265270407491  SaturateOnIntegerOverflow=on  OutDataTypeStr=Inherit: Same as input  ParamDataTypeStr=Inherit: Same as input
  b(38) : Gain  Gain=-0.038329320446368831  SaturateOnIntegerOverflow=on  OutDataTypeStr=Inherit: Same as input  ParamDataTypeStr=Inherit: Same as input
  b(39) : Gain  Gain=-0.0072704924773104732  SaturateOnIntegerOverflow=on  OutDataTypeStr=Inherit: Same as input  ParamDataTypeStr=Inherit: Same as input
  b(4) : Gain  Gain=-0.0032830177673830877  SaturateOnIntegerOverflow=on  OutDataTypeStr=Inherit: Same as input  ParamDataTypeStr=Inherit: Same as input
  b(40) : Gain  Gain=0.028242635943863115  SaturateOnIntegerOverflow=on  OutDataTypeStr=Inherit: Same as input  ParamDataTypeStr=Inherit: Same as input
  b(41) : Gain  Gain=0.0070602627960907726  SaturateOnIntegerOverflow=on  OutDataTypeStr=Inherit: Same as input  ParamDataTypeStr=Inherit: Same as input
  b(42) : Gain  Gain=-0.020867949959447688  SaturateOnIntegerOverflow=on  OutDataTypeStr=Inherit: Same as input  ParamDataTypeStr=Inherit: Same as input
  b(43) : Gain  Gain=-0.0065686388642668125  SaturateOnIntegerOverflow=on  OutDataTypeStr=Inherit: Same as input  ParamDataTypeStr=Inherit: Same as input
  b(44) : Gain  Gain=0.0151981830555213  SaturateOnIntegerOverflow=on  OutDataTypeStr=Inherit: Same as input  ParamDataTypeStr=Inherit: Same as input
  b(45) : Gain  Gain=0.005763535930488302  SaturateOnIntegerOverflow=on  OutDataTypeStr=Inherit: Same as input  ParamDataTypeStr=Inherit: Same as input
  b(46) : Gain  Gain=-0.011014879869749052  SaturateOnIntegerOverflow=on  OutDataTypeStr=Inherit: Same as input  ParamDataTypeStr=Inherit: Same as input
  b(47) : Gain  Gain=-0.0051172092513206528  SaturateOnIntegerOverflow=on  OutDataTypeStr=Inherit: Same as input  ParamDataTypeStr=Inherit: Same as input
  b(48) : Gain  Gain=0.0075034408734532838  SaturateOnIntegerOverflow=on  OutDataTypeStr=Inherit: Same as input  ParamDataTypeStr=Inherit: Same as input
  b(49) : Gain  Gain=0.0039498824016694816  SaturateOnIntegerOverflow=on  OutDataTypeStr=Inherit: Same as input  ParamDataTypeStr=Inherit: Same as input
  b(5) : Gain  Gain=0.0039854203993547575  SaturateOnIntegerOverflow=on  OutDataTypeStr=Inherit: Same as input  ParamDataTypeStr=Inherit: Same as input
  b(50) : Gain  Gain=-0.0056185919166622817  SaturateOnIntegerOverflow=on  OutDataTypeStr=Inherit: Same as input  ParamDataTypeStr=Inherit: Same as input
  b(51) : Gain  Gain=-0.0039854203993547575  SaturateOnIntegerOverflow=on  OutDataTypeStr=Inherit: Same as input  ParamDataTypeStr=Inherit: Same as input
  b(52) : Gain  Gain=0.0032830177673830877  SaturateOnIntegerOverflow=on  OutDataTypeStr=Inherit: Same as input  ParamDataTypeStr=Inherit: Same as input
  b(53) : Gain  Gain=0.0038948238157296179  SaturateOnIntegerOverflow=on  OutDataTypeStr=Inherit: Same as input  ParamDataTypeStr=Inherit: Same as input
  b(54) : Gain  Gain=-0.00017042943589110223  SaturateOnIntegerOverflow=on  OutDataTypeStr=Inherit: Same as input  ParamDataTypeStr=Inherit: Same as input
  b(55) : Gain  Gain=-0.0016485839041717864  SaturateOnIntegerOverflow=on  OutDataTypeStr=Inherit: Same as input  ParamDataTypeStr=Inherit: Same as input
  b(6) : Gain  Gain=0.0056185919166622817  SaturateOnIntegerOverflow=on  OutDataTypeStr=Inherit: Same as input  ParamDataTypeStr=Inherit: Same as input
  b(7) : Gain  Gain=-0.0039498824016694816  SaturateOnIntegerOverflow=on  OutDataTypeStr=Inherit: Same as input  ParamDataTypeStr=Inherit: Same as input
  b(8) : Gain  Gain=-0.0075034408734532838  SaturateOnIntegerOverflow=on  OutDataTypeStr=Inherit: Same as input  ParamDataTypeStr=Inherit: Same as input
  b(9) : Gain  Gain=0.0051172092513206528  SaturateOnIntegerOverflow=on  OutDataTypeStr=Inherit: Same as input  ParamDataTypeStr=Inherit: Same as input
  Output : Outport
  wires:
  Input/1 -> b(1)/1, BodyDelay2/1
  b(1)/1 -> BodyLSum2/2
  BodyDelay2/1 -> b(2)/1, BodyDelay3/1
  b(2)/1 -> BodyLSum2/1
  BodyLSum2/1 -> BodyLSum3/2
  BodyDelay3/1 -> b(3)/1, BodyDelay4/1
  b(3)/1 -> BodyLSum3/1
  BodyLSum3/1 -> BodyLSum4/2
  BodyDelay4/1 -> b(4)/1, BodyDelay5/1
  b(4)/1 -> BodyLSum4/1
  BodyLSum4/1 -> BodyLSum5/2
  BodyDelay5/1 -> b(5)/1, BodyDelay6/1
  b(5)/1 -> BodyLSum5/1
  BodyLSum5/1 -> BodyLSum6/2
  BodyDelay6/1 -> b(6)/1, BodyDelay7/1
  b(6)/1 -> BodyLSum6/1
  BodyLSum6/1 -> BodyLSum7/2
  BodyDelay7/1 -> b(7)/1, BodyDelay8/1
  b(7)/1 -> BodyLSum7/1
  BodyLSum7/1 -> BodyLSum8/2
  BodyDelay8/1 -> b(8)/1, BodyDelay9/1
  b(8)/1 -> BodyLSum8/1
  BodyLSum8/1 -> BodyLSum9/2
  BodyDelay9/1 -> b(9)/1, BodyDelay10/1
  b(9)/1 -> BodyLSum9/1
  BodyLSum9/1 -> BodyLSum10/2
  BodyDelay10/1 -> b(10)/1, BodyDelay11/1
  b(10)/1 -> BodyLSum10/1
  BodyLSum10/1 -> BodyLSum11/2
  BodyDelay11/1 -> b(11)/1, BodyDelay12/1
  b(11)/1 -> BodyLSum11/1
  BodyLSum11/1 -> BodyLSum12/2
  BodyDelay12/1 -> b(12)/1, BodyDelay13/1
  b(12)/1 -> BodyLSum12/1
  BodyLSum12/1 -> BodyLSum13/2
  BodyDelay13/1 -> b(13)/1, BodyDelay14/1
  b(13)/1 -> BodyLSum13/1
  BodyLSum13/1 -> BodyLSum14/2
  BodyDelay14/1 -> b(14)/1, BodyDelay15/1
  b(14)/1 -> BodyLSum14/1
  BodyLSum14/1 -> BodyLSum15/2
  BodyDelay15/1 -> b(15)/1, BodyDelay16/1
  b(15)/1 -> BodyLSum15/1
  BodyLSum15/1 -> BodyLSum16/2
  BodyDelay16/1 -> b(16)/1, BodyDelay17/1
  b(16)/1 -> BodyLSum16/1
  BodyLSum16/1 -> BodyLSum17/2
  BodyDelay17/1 -> b(17)/1, BodyDelay18/1
  b(17)/1 -> BodyLSum17/1
  BodyLSum17/1 -> BodyLSum18/2
  BodyDelay18/1 -> b(18)/1, BodyDelay19/1
  b(18)/1 -> BodyLSum18/1
  BodyLSum18/1 -> BodyLSum19/2
  BodyDelay19/1 -> b(19)/1, BodyDelay20/1
  b(19)/1 -> BodyLSum19/1
  BodyLSum19/1 -> BodyLSum20/2
  BodyDelay20/1 -> b(20)/1, BodyDelay21/1
  b(20)/1 -> BodyLSum20/1
  BodyLSum20/1 -> BodyLSum21/2
  BodyDelay21/1 -> b(21)/1, BodyDelay22/1
  b(21)/1 -> BodyLSum21/1
  BodyLSum21/1 -> BodyLSum22/2
  BodyDelay22/1 -> b(22)/1, BodyDelay23/1
  b(22)/1 -> BodyLSum22/1
  BodyLSum22/1 -> BodyLSum23/2
  BodyDelay23/1 -> b(23)/1, BodyDelay24/1
  b(23)/1 -> BodyLSum23/1
  BodyLSum23/1 -> BodyLSum24/2
  BodyDelay24/1 -> b(24)/1, BodyDelay25/1
  b(24)/1 -> BodyLSum24/1
  BodyLSum24/1 -> BodyLSum25/2
  BodyDelay25/1 -> b(25)/1, BodyDelay26/1
  b(25)/1 -> BodyLSum25/1
  BodyLSum25/1 -> BodyLSum26/2
  BodyDelay26/1 -> b(26)/1, BodyDelay27/1
  b(26)/1 -> BodyLSum26/1
  BodyLSum26/1 -> BodyLSum27/2
  BodyDelay27/1 -> b(27)/1, BodyDelay29/1
  b(27)/1 -> BodyLSum27/1
  BodyLSum27/1 -> BodyLSum29/2
  BodyDelay29/1 -> b(29)/1, BodyDelay30/1
  b(29)/1 -> BodyLSum29/1
  BodyLSum29/1 -> BodyLSum30/2
  BodyDelay30/1 -> b(30)/1, BodyDelay31/1
  b(30)/1 -> BodyLSum30/1
  BodyLSum30/1 -> BodyLSum31/2
  BodyDelay31/1 -> b(31)/1, BodyDelay32/1
  b(31)/1 -> BodyLSum31/1
  BodyLSum31/1 -> BodyLSum32/2
  BodyDelay32/1 -> b(32)/1, BodyDelay33/1
  b(32)/1 -> BodyLSum32/1
  BodyLSum32/1 -> BodyLSum33/2
  BodyDelay33/1 -> b(33)/1, BodyDelay34/1
  b(33)/1 -> BodyLSum33/1
  BodyLSum33/1 -> BodyLSum34/2
  BodyDelay34/1 -> b(34)/1, BodyDelay35/1
  b(34)/1 -> BodyLSum34/1
  BodyLSum34/1 -> BodyLSum35/2
  BodyDelay35/1 -> b(35)/1, BodyDelay36/1
  b(35)/1 -> BodyLSum35/1
  BodyLSum35/1 -> BodyLSum36/2
  BodyDelay36/1 -> b(36)/1, BodyDelay37/1
  b(36)/1 -> BodyLSum36/1
  BodyLSum36/1 -> BodyLSum37/2
  BodyDelay37/1 -> b(37)/1, BodyDelay38/1
  b(37)/1 -> BodyLSum37/1
  BodyLSum37/1 -> BodyLSum38/2
  BodyDelay38/1 -> b(38)/1, BodyDelay39/1
  b(38)/1 -> BodyLSum38/1
  BodyLSum38/1 -> BodyLSum39/2
  BodyDelay39/1 -> b(39)/1, BodyDelay40/1
  b(39)/1 -> BodyLSum39/1
  BodyLSum39/1 -> BodyLSum40/2
  BodyDelay40/1 -> b(40)/1, BodyDelay41/1
  b(40)/1 -> BodyLSum40/1
  BodyLSum40/1 -> BodyLSum41/2
  BodyDelay41/1 -> b(41)/1, BodyDelay42/1
  b(41)/1 -> BodyLSum41/1
  BodyLSum41/1 -> BodyLSum42/2
  BodyDelay42/1 -> b(42)/1, BodyDelay43/1
  b(42)/1 -> BodyLSum42/1
  BodyLSum42/1 -> BodyLSum43/2
  BodyDelay43/1 -> b(43)/1, BodyDelay44/1
  b(43)/1 -> BodyLSum43/1
  BodyLSum43/1 -> BodyLSum44/2
  BodyDelay44/1 -> b(44)/1, BodyDelay45/1
  b(44)/1 -> BodyLSum44/1
  BodyLSum44/1 -> BodyLSum45/2
  BodyDelay45/1 -> b(45)/1, BodyDelay46/1
  b(45)/1 -> BodyLSum45/1
  BodyLSum45/1 -> BodyLSum46/2
  BodyDelay46/1 -> b(46)/1, BodyDelay47/1
  b(46)/1 -> BodyLSum46/1
  BodyLSum46/1 -> BodyLSum47/2
  BodyDelay47/1 -> b(47)/1, BodyDelay48/1
  b(47)/1 -> BodyLSum47/1
  BodyLSum47/1 -> BodyLSum48/2
  BodyDelay48/1 -> b(48)/1, BodyDelay49/1
  b(48)/1 -> BodyLSum48/1
  BodyLSum48/1 -> BodyLSum49/2
  BodyDelay49/1 -> b(49)/1, BodyDelay50/1
  b(49)/1 -> BodyLSum49/1
  BodyLSum49/1 -> BodyLSum50/2
  BodyDelay50/1 -> b(50)/1, BodyDelay51/1
  b(50)/1 -> BodyLSum50/1
  BodyLSum50/1 -> BodyLSum51/2
  BodyDelay51/1 -> b(51)/1, BodyDelay52/1
  b(51)/1 -> BodyLSum51/1
  BodyLSum51/1 -> BodyLSum52/2
  BodyDelay52/1 -> b(52)/1, BodyDelay53/1
  b(52)/1 -> BodyLSum52/1
  BodyLSum52/1 -> BodyLSum53/2
  BodyDelay53/1 -> b(53)/1, BodyDelay54/1
  b(53)/1 -> BodyLSum53/1
  BodyLSum53/1 -> BodyLSum54/2
  BodyDelay54/1 -> b(54)/1, BodyDelay55/1
  b(54)/1 -> BodyLSum54/1
  BodyLSum54/1 -> BodyLSum55/1
  BodyDelay55/1 -> b(55)/1
  b(55)/1 -> BodyLSum55/2
  BodyLSum55/1 -> Output/1

== system microgridbelbic/Subsystem1/Subsystem/array1/Solar/Subsystem1 ==
  In1 : Inport
  Current Measurement : powerlib/Measurements/Current Measurement  PhasorSimulation=off  OutputType=Complex  PSBequivalent=0
      settings: SourceProductName=Simscape Electrical
  Insolation to current gain : Gain  Gain=8.01/1000  SampleTime=20e-6
  Scope : Scope
  Scope1 : Scope
  Subsystem : Subsystem
  Voltage Measurement : powerlib/Measurements/Voltage Measurement  PhasorSimulation=off  OutputType=Complex  PSBequivalent=0
      settings: SourceProductName=Simscape Electrical
  + : PMIOPort  Side=Right
  - : PMIOPort  Port=2  Side=Right
  wires:
  Current Measurement/1 -> Scope1/1
  Voltage Measurement/1 -> Scope/1
  In1/1 -> Insolation to current gain/1
  Insolation to current gain/1 -> Subsystem/1(irrad)
  connections:
  Current Measurement/RConn1 -- +/RConn1
  Voltage Measurement/LConn2 -- Subsystem/RConn2 -- -/RConn1
  Current Measurement/LConn1 -- Subsystem/RConn1 -- Voltage Measurement/LConn1

== system microgridbelbic/Subsystem1/Subsystem/array1/Solar/Subsystem5 ==
  In1 : Inport
  Current Measurement : powerlib/Measurements/Current Measurement  PhasorSimulation=off  OutputType=Complex  PSBequivalent=0
      settings: SourceProductName=Simscape Electrical
  Insolation to current gain : Gain  Gain=8.01/1000  SampleTime=20e-6
  Scope : Scope
  Scope1 : Scope
  Subsystem : Subsystem
  Voltage Measurement : powerlib/Measurements/Voltage Measurement  PhasorSimulation=off  OutputType=Complex  PSBequivalent=0
      settings: SourceProductName=Simscape Electrical
  + : PMIOPort  Side=Right
  - : PMIOPort  Port=2  Side=Right
  wires:
  Insolation to current gain/1 -> Subsystem/1(irrad)
  In1/1 -> Insolation to current gain/1
  Voltage Measurement/1 -> Scope/1
  Current Measurement/1 -> Scope1/1
  connections:
  Voltage Measurement/LConn1 -- Subsystem/RConn1 -- Current Measurement/LConn1
  -/RConn1 -- Subsystem/RConn2 -- Voltage Measurement/LConn2
  Current Measurement/RConn1 -- +/RConn1

== system microgridbelbic/Subsystem1/Subsystem/array6/Solar/11= Vmpp=336V, Voc=406V ==
  In1 : Inport
  Current Measurement : powerlib/Measurements/Current Measurement  PhasorSimulation=off  OutputType=Complex  PSBequivalent=0
      settings: SourceProductName=Simscape Electrical
  Insolation to current gain : Gain  Gain=8.01/1000  SampleTime=20e-6
  Scope : Scope
  Scope1 : Scope
  Subsystem : Subsystem
  Voltage Measurement : powerlib/Measurements/Voltage Measurement  PhasorSimulation=off  OutputType=Complex  PSBequivalent=0
      settings: SourceProductName=Simscape Electrical
  + : PMIOPort  Side=Right
  - : PMIOPort  Port=2  Side=Right
  wires:
  Current Measurement/1 -> Scope1/1
  Voltage Measurement/1 -> Scope/1
  In1/1 -> Insolation to current gain/1
  Insolation to current gain/1 -> Subsystem/1(irrad)
  connections:
  Current Measurement/RConn1 -- +/RConn1
  Voltage Measurement/LConn2 -- Subsystem/RConn2 -- -/RConn1
  Current Measurement/LConn1 -- Subsystem/RConn1 -- Voltage Measurement/LConn1

== system microgridbelbic/Subsystem1/Subsystem/array6/Solar/11=336V, 406 V ==
  In1 : Inport
  Current Measurement : powerlib/Measurements/Current Measurement  PhasorSimulation=off  OutputType=Complex  PSBequivalent=0
      settings: SourceProductName=Simscape Electrical
  Insolation to current gain : Gain  Gain=8.01/1000  SampleTime=20e-6
  Scope : Scope
  Scope1 : Scope
  Subsystem : Subsystem
  Voltage Measurement : powerlib/Measurements/Voltage Measurement  PhasorSimulation=off  OutputType=Complex  PSBequivalent=0
      settings: SourceProductName=Simscape Electrical
  + : PMIOPort  Side=Right
  - : PMIOPort  Port=2  Side=Right
  wires:
  Insolation to current gain/1 -> Subsystem/1(irrad)
  In1/1 -> Insolation to current gain/1
  Voltage Measurement/1 -> Scope/1
  Current Measurement/1 -> Scope1/1
  connections:
  Voltage Measurement/LConn1 -- Subsystem/RConn1 -- Current Measurement/LConn1
  -/RConn1 -- Subsystem/RConn2 -- Voltage Measurement/LConn2
  Current Measurement/RConn1 -- +/RConn1
